simulink model "Carla"  (R2022a)
settings: Solver=VariableStepAuto  StartTime=0.0  StopTime=inf  RelTol=1e-3
libraries: visionsinks x4
settings Model: Creator=darks  LastModifiedBy=cc
settings SolverCC: AlgebraicLoopSolver=TrustRegion
settings DebuggingCC: UnconnectedInputMsg=warning  UnconnectedOutputMsg=warning  UnconnectedLineMsg=warning  SFMachineParentedDataDiag=warning
settings SFSimCC: CustomCodeUndefinedFunction=UseInterfaceOnly

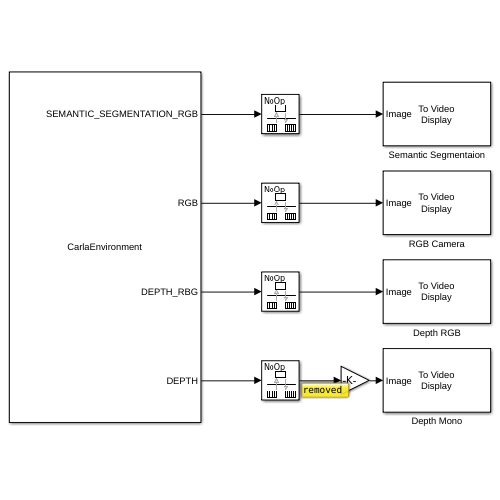
[thumbnail: Simulink's stored preview of the top-level diagram]
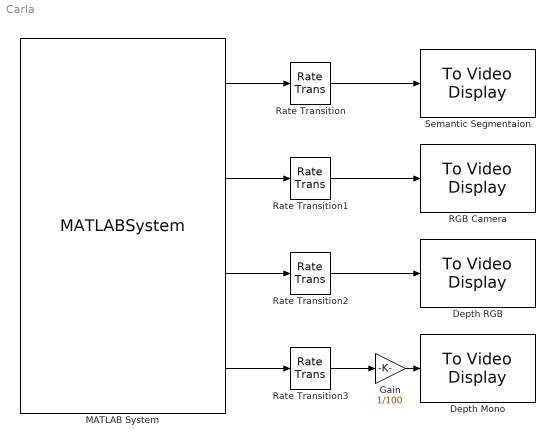
== system Carla ==
  Depth Mono : visionsinks/To Video Display  windowSizeMode=Normal  openAtMdlStart=off  fullScreen=off  videoWindowX=4414  videoWindowY=698  saveWindowSize=off  videoWindowWidth=498  videoWindowHeight=397  inputColorFormat=RGB  inputType=Obsolete  imagePorts=One multidimensional signal  OutputDevice=On-screen video monitor  dataOrg=Column-major  isWindowOpen=off
  Depth RGB : visionsinks/To Video Display  windowSizeMode=Normal  openAtMdlStart=off  fullScreen=off  videoWindowX=4245  videoWindowY=389  saveWindowSize=off  videoWindowWidth=473  videoWindowHeight=270  inputColorFormat=RGB  inputType=Obsolete  imagePorts=One multidimensional signal  OutputDevice=On-screen video monitor  dataOrg=Column-major  isWindowOpen=off
  Gain : Gain  Gain=1/100
  MATLAB System : MATLABSystem  System=CarlaEnvironment  SimulateUsing=Interpreted execution
      mask Type: CarlaEnvironment
      mask Display:
      | disp('CarlaEnvironment');
      | port_label('output',1,'SEMANTIC_SEGMENTATION_RGB');
      | port_label('output',2,'RGB');
      | port_label('output',3,'DEPTH_RBG');
      | port_label('output',4,'DEPTH');
  RGB Camera : visionsinks/To Video Display  windowSizeMode=Normal  openAtMdlStart=off  fullScreen=off  videoWindowX=3832  videoWindowY=699  saveWindowSize=off  videoWindowWidth=564  videoWindowHeight=356  inputColorFormat=RGB  inputType=Obsolete  imagePorts=One multidimensional signal  OutputDevice=On-screen video monitor  dataOrg=Column-major  isWindowOpen=off
  Rate Transition{,1..3} (4 alike) : RateTransition  OutPortSampleTime=.1
  Semantic Segmentaion : visionsinks/To Video Display  windowSizeMode=Normal  openAtMdlStart=off  fullScreen=off  videoWindowX=10  videoWindowY=8  saveWindowSize=off  videoWindowWidth=404  videoWindowHeight=269  inputColorFormat=RGB  inputType=Obsolete  imagePorts=One multidimensional signal  OutputDevice=On-screen video monitor  dataOrg=Column-major  isWindowOpen=off
  wires:
  Rate Transition/1 -> Semantic Segmentaion/1
  MATLAB System/1 -> Rate Transition/1
  MATLAB System/2 -> Rate Transition1/1
  Rate Transition1/1 -> RGB Camera/1
  Rate Transition2/1 -> Depth RGB/1
  MATLAB System/3 -> Rate Transition2/1
  MATLAB System/4 -> Rate Transition3/1
  Rate Transition3/1 -> Gain/1
  Gain/1 -> Depth Mono/1
